simulink model "Open_Closed_Loopes_WithoutController"  (R2022b)
settings: Solver=VariableStepAuto  StartTime=0.0  StopTime=20  MaxStep=1e-3  RelTol=1e-3
settings Model: Creator=Mo_7atem  LastModifiedBy=Mo_7atem

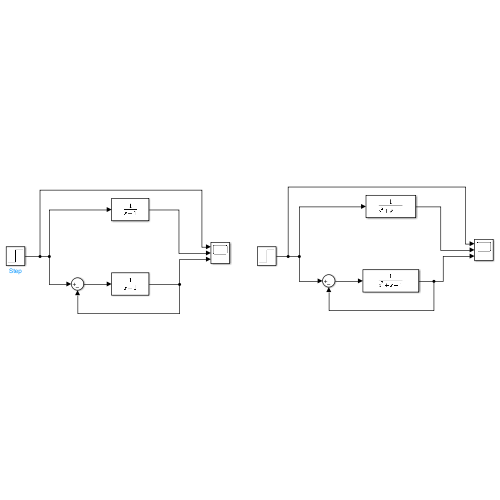
[thumbnail: Simulink's stored preview of the top-level diagram]
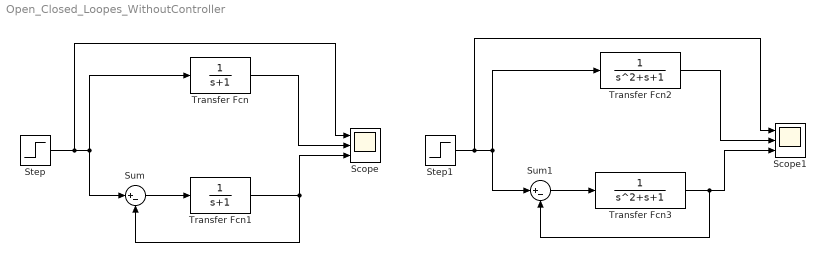
== system Open_Closed_Loopes_WithoutController ==
  Scope : Scope  NumInputPorts=3
  Scope1 : Scope  NumInputPorts=3
  Step : Step  SampleTime=0
  Step1 : Step  SampleTime=0
  Sum : Sum  Inputs=|+-
  Sum1 : Sum  Inputs=|+-
  Transfer Fcn : TransferFcn  Denominator=[1 1]
  Transfer Fcn1 : TransferFcn  Denominator=[1 1]
  Transfer Fcn2 : TransferFcn  Denominator=[1 1 1]
  Transfer Fcn3 : TransferFcn  Denominator=[1 1 1]
  wires:
  Transfer Fcn/1 -> Scope/2
  Sum/1 -> Transfer Fcn1/1
  Transfer Fcn1/1 -> Scope/3, Sum/2
  Step/1 -> Scope/1, Transfer Fcn/1, Sum/1
  Transfer Fcn3/1 -> Scope1/3, Sum1/2
  Step1/1 -> Transfer Fcn2/1, Sum1/1, Scope1/1
  Sum1/1 -> Transfer Fcn3/1
  Transfer Fcn2/1 -> Scope1/2
